simulink model "mbd"  (R2022b)
settings: Solver=ode45  StartTime=0.0  StopTime=10.0  FixedStep=Ts  MaxStep=Ts  RelTol=1e-3
PreLoadFcn:
  | preload
  | conf
InitFcn:
  | plant
  | control
values from neighbouring files (symbols this model uses):
  A1 = [0 0   1 0 ... (first row only)    [plant.m]
  A2 = [0   1 ... (first row only)    [plant.m]
  B1 = [0 0 ... (first row only)    [plant.m]
  B2 = [0    0 ... (first row only)    [plant.m]
  C1 = eye(4)    [plant.m]
  C2 = eye(2)    [plant.m]
  D1 = zeros(4, 2)    [plant.m]
  D2 = zeros(2)    [plant.m]
  K = lqrd(s3.A, s3.B, QQ, RR, Ts)    [control.m]    (also in plant.m = W / (2 * R) * alpha)
  K_PWM = 8.087    [params.m]
  Psi0 = 0.01    [params.m]
  R = 0.027    [params.m]
  W = 0.105    [params.m]
undefined symbols (not defined in the file or in its folder): DiscIntNeverNeededParam
libraries: simulink_extras x2, simulink x1
settings Model: Creator=Viktor  LastModifiedBy=Viktor
settings SolverCC: ZeroCrossAlgorithm=Adaptive

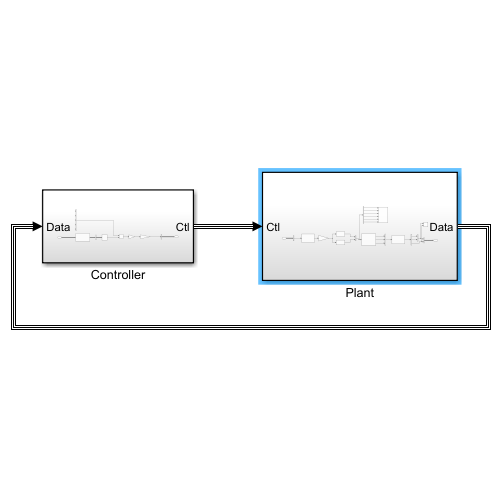
[thumbnail: Simulink's stored preview of the top-level diagram]
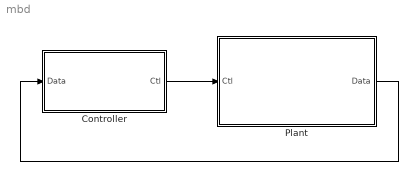
== system mbd ==
  Controller : Subsystem
  Plant : Subsystem
  wires:
  Controller/1(Ctl) -> Plant/1(Ctl)
  Plant/1(Data) -> Controller/1(Data)

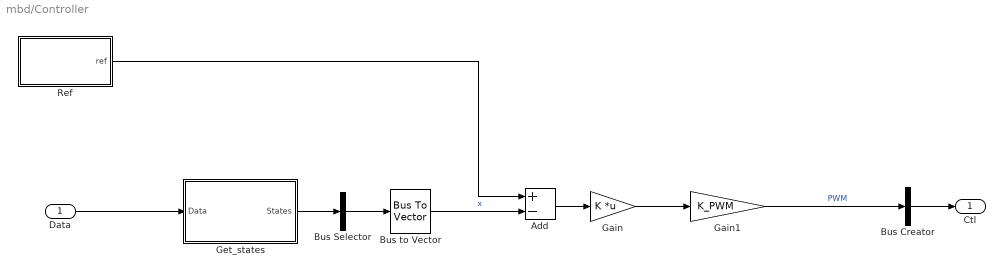
== system mbd/Controller ==
  Data : Inport
  Add : Sum  Inputs=+-
  Bus Creator : BusCreator  Inputs=1  OutDataTypeStr=Bus: Ctl
  Bus Selector : BusSelector  OutputSignals=theta_int,theta,psi,theta_dot,psi_dot  OutputAsBus=on
  Bus to Vector : BusToVector
  Gain : Gain  Gain=K  Multiplication=Matrix(K*u)
  Gain1 : Gain  Gain=K_PWM
  Get_states : Subsystem
  Ref : Subsystem
  Ctl : Outport
  wires:
  Bus Creator/1 -> Ctl/1
  Data/1 -> Get_states/1(Data)
  Get_states/1(States) -> Bus Selector/1
  Bus Selector/1 -> Bus to Vector/1
  Bus to Vector/1 -> Add/2  "x"
  Ref/1(ref) -> Add/1
  Gain1/1 -> Bus Creator/1  "PWM"
  Add/1 -> Gain/1
  Gain/1 -> Gain1/1

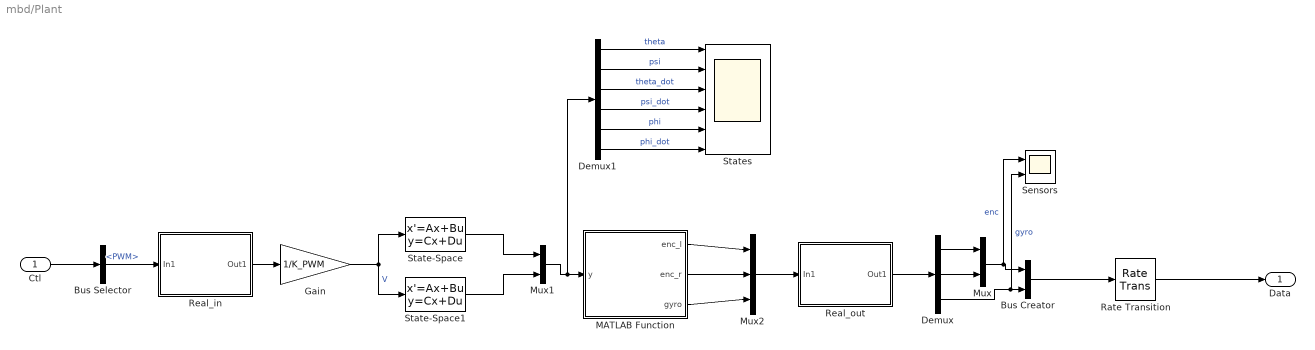
== system mbd/Plant ==
  Ctl : Inport
  Bus Creator : BusCreator  Inputs=2  OutDataTypeStr=Bus: Data
  Bus Selector : BusSelector  OutputSignals=PWM
  Demux : Demux  Outputs=3
  Demux1 : Demux  Outputs=6
  Gain : Gain  Gain=1/K_PWM
  MATLAB Function : MATLAB Function  TreatAsAtomicUnit=on
  Mux : Mux  Inputs=2
  Mux1 : Mux  Inputs=2
  Mux2 : Mux  Inputs=3
  Rate Transition : RateTransition  OutPortSampleTime=Ts
  Real_in : Subsystem  Variant=on  VariantControl=Choice
  Real_out : Subsystem  Variant=on  VariantControl=Choice
  Sensors : Scope  NumInputPorts=2
  State-Space : StateSpace  A=A1  B=B1  C=C1  D=D1  InitialCondition=[0 Psi0 0 0]
  State-Space1 : StateSpace  A=A2  B=B2  C=C2  D=D2  InitialCondition=0
  States : Scope  NumInputPorts=6
  Data : Outport
  wires:
  State-Space/1 -> Mux1/1
  Real_in/1(Out1) -> Gain/1
  MATLAB Function/1(enc_l) -> Mux2/1
  Mux2/1 -> Real_out/1(In1)
  MATLAB Function/3(gyro) -> Mux2/3
  Gain/1 -> State-Space/1, State-Space1/1  "V"
  Mux1/1 -> Demux1/1, MATLAB Function/1(y)
  State-Space1/1 -> Mux1/2
  MATLAB Function/2(enc_r) -> Mux2/2
  Real_out/1(Out1) -> Demux/1
  Demux/2 -> Mux/2
  Demux/1 -> Mux/1
  Demux/3 -> Bus Creator/2, Sensors/2  "gyro"
  Mux/1 -> Sensors/1, Bus Creator/1  "enc"
  Bus Creator/1 -> Rate Transition/1
  Ctl/1 -> Bus Selector/1
  Bus Selector/1 -> Real_in/1(In1)  "<PWM>"
  Demux1/1 -> States/1  "theta"
  Demux1/2 -> States/2  "psi"
  Demux1/3 -> States/3  "theta_dot"
  Demux1/4 -> States/4  "psi_dot"
  Demux1/5 -> States/5  "phi"
  Demux1/6 -> States/6  "phi_dot"
  Rate Transition/1 -> Data/1

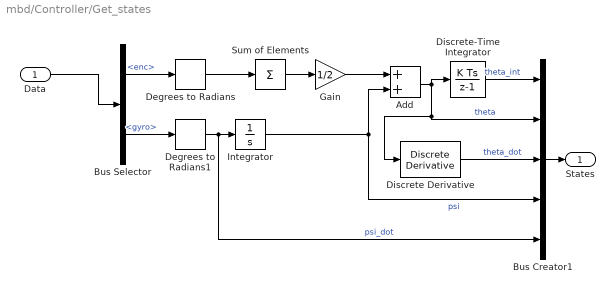
== system mbd/Controller/Get_states ==
  Data : Inport
  Add : Sum
  Bus Creator1 : BusCreator  Inputs=5
  Bus Selector : BusSelector  OutputSignals=enc,gyro
  Degrees to Radians : simulink_extras/Transformations/Degrees to Radians
  Degrees to Radians1 : simulink_extras/Transformations/Degrees to Radians
  Discrete Derivative : simulink/Discrete/Discrete Derivative  gainval=1.0  ICPrevScaledInput=0.0  OutMin=[]  OutMax=[]  OutDataType=fixdt(1, 16)  OutScaling=2^-10  DoSatur=off
  Discrete-Time Integrator : DiscreteIntegrator  SampleTime=-1  ICPrevOutput=DiscIntNeverNeededParam  ICPrevScaledInput=DiscIntNeverNeededParam
  Gain : Gain  Gain=1/2
  Integrator : Integrator
  Sum of Elements : Sum  Inputs=+
  States : Outport
  wires:
  Data/1 -> Bus Selector/1
  Sum of Elements/1 -> Gain/1
  Bus Selector/2 -> Degrees to Radians1/1  "<gyro>"
  Integrator/1 -> Bus Creator1/4, Add/2  "psi"
  Bus Creator1/1 -> States/1
  Add/1 -> Discrete-Time Integrator/1, Discrete Derivative/1, Bus Creator1/2  "theta"
  Degrees to Radians1/1 -> Bus Creator1/5, Integrator/1  "psi_dot"
  Gain/1 -> Add/1
  Bus Selector/1 -> Degrees to Radians/1  "<enc>"
  Degrees to Radians/1 -> Sum of Elements/1
  Discrete-Time Integrator/1 -> Bus Creator1/1  "theta_int"
  Discrete Derivative/1 -> Bus Creator1/3  "theta_dot"

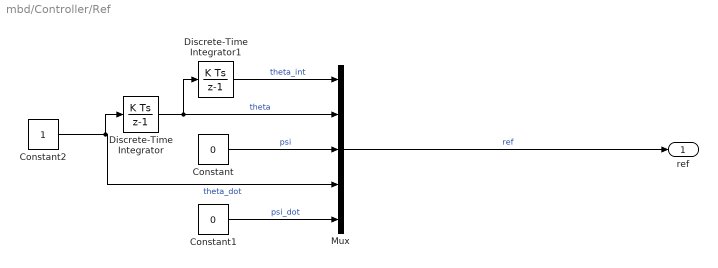
== system mbd/Controller/Ref ==
  Constant : Constant  Value=0
  Constant1 : Constant  Value=0
  Constant2 : Constant
  Discrete-Time Integrator : DiscreteIntegrator  SampleTime=-1  ICPrevOutput=DiscIntNeverNeededParam  ICPrevScaledInput=DiscIntNeverNeededParam
  Discrete-Time Integrator1 : DiscreteIntegrator  SampleTime=-1  ICPrevOutput=DiscIntNeverNeededParam  ICPrevScaledInput=DiscIntNeverNeededParam
  Mux : Mux  Inputs=5
  ref : Outport
  wires:
  Discrete-Time Integrator1/1 -> Mux/1  "theta_int"
  Discrete-Time Integrator/1 -> Discrete-Time Integrator1/1, Mux/2  "theta"
  Constant1/1 -> Mux/5  "psi_dot"
  Constant2/1 -> Discrete-Time Integrator/1, Mux/4  "theta_dot"
  Constant/1 -> Mux/3  "psi"
  Mux/1 -> ref/1  "ref"

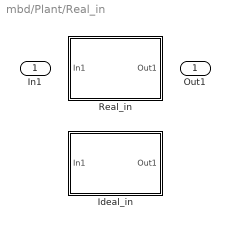
== system mbd/Plant/Real_in ==
  In1 : Inport
  Ideal_in : Subsystem  VariantControl=(default)
  Real_in : Subsystem  VariantControl=real_model == 1
  Out1 : Outport

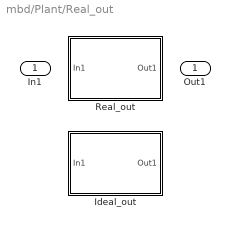
== system mbd/Plant/Real_out ==
  In1 : Inport
  Ideal_out : Subsystem  VariantControl=(default)
  Real_out : Subsystem  VariantControl=real_model == 1
  Out1 : Outport

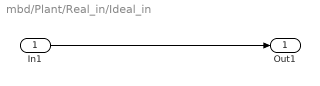
== system mbd/Plant/Real_in/Ideal_in ==
  In1 : Inport
  Out1 : Outport
  wires:
  In1/1 -> Out1/1

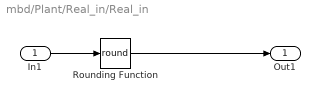
== system mbd/Plant/Real_in/Real_in ==
  In1 : Inport
  Rounding Function : Rounding  Operator=round
  Out1 : Outport
  wires:
  In1/1 -> Rounding Function/1
  Rounding Function/1 -> Out1/1

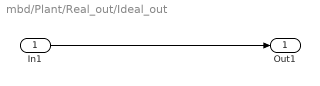
== system mbd/Plant/Real_out/Ideal_out ==
  In1 : Inport
  Out1 : Outport
  wires:
  In1/1 -> Out1/1

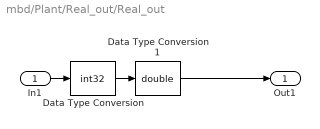
== system mbd/Plant/Real_out/Real_out ==
  In1 : Inport
  Data Type Conversion : DataTypeConversion  OutDataTypeStr=int32  SaturateOnIntegerOverflow=off  RndMeth=Floor
  Data Type Conversion1 : DataTypeConversion  OutDataTypeStr=double  SaturateOnIntegerOverflow=off  RndMeth=Floor
  Out1 : Outport
  wires:
  Data Type Conversion/1 -> Data Type Conversion1/1
  In1/1 -> Data Type Conversion/1
  Data Type Conversion1/1 -> Out1/1

== matlab function mbd/Plant/MATLAB Function ==
  data: y input; enc_l output; enc_r output; gyro output; R parameter; W parameter
function [enc_l, enc_r, gyro] = sensors(y, R, W)
enc_l = rad2deg(y(1) - W/R/2 * y(5) - y(2));
enc_r = rad2deg(y(1) + W/R/2 * y(5) - y(2));
gyro = rad2deg(y(4));
